simulink model "SF103A_MotRefMdl"  (R2013b)
settings: Solver=FixedStepDiscrete  StartTime=0.0  StopTime=2  FixedStep=.002  RelTol=1e-3
values from neighbouring files (symbols this model uses):
  ARCHGLBPRM_2MILLISEC_SEC_F32 = DataDict.Constant    [SF103A_MotRefMdl_DataDict.m]
  ARCHGLBPRM_2OVERSQRT3_ULS_F32 = DataDict.Constant    [SF103A_MotRefMdl_DataDict.m]
  ARCHGLBPRM_2PI_ULS_F32 = DataDict.Constant    [SF103A_MotRefMdl_DataDict.m]
  ARCHGLBPRM_4OVERSQRT3_ULS_F32 = DataDict.Constant    [SF103A_MotRefMdl_DataDict.m]
  ARCHGLBPRM_5PIOVER4_ULS_F32 = DataDict.Constant    [SF103A_MotRefMdl_DataDict.m]
  ARCHGLBPRM_FLOATZEROTHD_ULS_F32 = DataDict.Constant    [SF103A_MotRefMdl_DataDict.m]
  ARCHGLBPRM_HALFSQRT3_ULS_F32 = DataDict.Constant    [SF103A_MotRefMdl_DataDict.m]
  ARCHGLBPRM_PI_ULS_F32 = DataDict.Constant    [SF103A_MotRefMdl_DataDict.m]
  MotRefMdlCurrDaxBoostGain = DataDict.Calibration    [SF103A_MotRefMdl_DataDict.m]
  MotRefMdlCurrDaxQaxRefDelta = DataDict.Calibration    [SF103A_MotRefMdl_DataDict.m]
  MotRefMdlCurrItrnTolr = DataDict.Calibration    [SF103A_MotRefMdl_DataDict.m]
  MotRefMdlFbCtrlDi = DataDict.Calibration    [SF103A_MotRefMdl_DataDict.m]
  MotRefMdlIvtrDeadTiBrdgVltgSca = DataDict.Calibration    [SF103A_MotRefMdl_DataDict.m]
  MotRefMdlMinCurrItrnLim = DataDict.Calibration    [SF103A_MotRefMdl_DataDict.m]
  MotRefMdlMotCurrDaxMaxSca = DataDict.Calibration    [SF103A_MotRefMdl_DataDict.m]
  MotRefMdlMotVltgDerivtvTiCon = DataDict.Calibration    [SF103A_MotRefMdl_DataDict.m]
  MotRefMdlRefLocnItrnLim = DataDict.Calibration    [SF103A_MotRefMdl_DataDict.m]
  MotRefMdlTqItrnLim = DataDict.Calibration    [SF103A_MotRefMdl_DataDict.m]
  MotRefMdlTqItrnTolr = DataDict.Calibration    [SF103A_MotRefMdl_DataDict.m]
  MotRefMdlVltgModDynCmpEna = DataDict.Calibration    [SF103A_MotRefMdl_DataDict.m]
  MotRefMdlVltgOverRThdSca = DataDict.Calibration    [SF103A_MotRefMdl_DataDict.m]
  SysGlbPrmMotPoleCnt = DataDict.ImprtdCal    [SF103A_MotRefMdl_DataDict.m]
undefined symbols (not defined in the file or in its folder): MotQuad1
libraries: NxtrLim x19, simulink x4, LnrIntrpn x3, Fil x2, NxtrAbslt x2, FixdToFloat x2, FloatToFixd x2, NxtrMath x1
(part 6 of 7)

== system SF103A_MotRefMdl/MotRefMdl/MotRefMdlPer1/DAxisCurrentBoost/If Action Subsystem/If Action Subsystem ==
  note: Rqmts: "BoostAmount"
  note: in requirments module: "VoltageMargin"
  note: Calculate CurrQax
  VRDelta : Inport  RequirementInfo={} %GIDa_629b2140_8cdd_4a04_85a5_53862d241c2d
  InterCalcns : Inport  RequirementInfo={} %GIDa_7ac02062_35f9_44f2_b401_9b07d57448af  Port=2
  CurrDaxMin : Inport  Port=3
  MotTqCmdLimd : Inport  RequirementInfo={} %GIDa_90d50d19_7197_48de_abc9_fa58816f1132  Port=4
  CurrDaxAtPeakTq : Inport  RequirementInfo={} %GIDa_cec05ccb_ae96_4c57_ae99_442dcea898ad  Port=5
  Action Port : ActionPort  ActionType=then
  Abs : Abs  RequirementInfo={'linktype_rmi_doors' '0000bb42 (/E-STEER Core/SubSystem Specifications/Application Functions/SF99/SF103A Motor Reference Model)' '#SF103A_150' 'true' 'REQ:SF103A_150' '' ; 'linktype_rmi_doors' '0000bb42 (/E-STEER Core/SubSystem Specifications/Application Functions/SF99/SF103A Motor Reference Model)' '#SF103A_151' 'true' 'REQ:SF103A_151' '' } %GIDa_3ad1a6bf_5535_4d0e_9aec_c451eb14e8f9
  Add : Sum  RequirementInfo={'linktype_rmi_doors' '0000bb42 (/E-STEER Core/SubSystem Specifications/Application Functions/SF99/SF103A Motor Reference Model)' '#SF103A_154' 'true' 'REQ:SF103A_154' '' } %GIDa_4db111d5_ebda_406f_9d3c_05162b6916bd
  Bus Selector : BusSelector  RequirementInfo={} %GIDa_2a56c463_8bdd_40e7_a9f9_22e566269336  OutputSignals=Ke_VoltPerRadPerSec,RelncTqCoeff_Henry_f32
  Constant1 : Constant  RequirementInfo={'linktype_rmi_doors' '0000bb42 (/E-STEER Core/SubSystem Specifications/Application Functions/SF99/SF103A Motor Reference Model)' '#SF103A_151' 'true' 'REQ:SF103A_151' '' } %GIDa_e17e5b1c_bcf6_46d0_81a3_c3a5d046727d  Value=MotRefMdlCurrDaxBoostGain
  CopyRight2 : Subsystem  Description=|  mask(Copyright Information){none=on}
      | Copyright info block.                                               
      |                                                                     
      | Place copyright information at the top of every subsystem in design.
      mask prompts: none "No parameters"
      mask help: Place copyright information at the top of every subsystem in design.
      mask Display:
      | NxtrConf = 'Nexteer Confidential';
      | 
      | sys = bdroot; %handle for the current model ("system")
      | first = get_param(sys,'Created');
      | first = first(end-3:end);  %year is last four digits
      | 
      | last = get_param(sys,'LastModifiedDate');
      | if isempty(last)
      |     last = datestr(now,'yyyy');
      | else
      |     last = last(end-3:end);
      | end
      | 
      | if strcmp(first,last)
      |     fprintf('%s -- Copyright %s Nexteer',NxtrConf,first)
      | else
      |     fprintf('%s -- %s%s- %s Nexteer',NxtrConf,char(169),first,last)
      | end
  Divide : Product  RequirementInfo={'linktype_rmi_doors' '0000bb42 (/E-STEER Core/SubSystem Specifications/Application Functions/SF99/SF103A Motor Reference Model)' '#SF103A_154' 'true' 'REQ:SF103A_154' '' } %GIDa_ca7e6ec7_86d7_4da8_a1df_b3e0eff68209  Inputs=*/
  FixdToFloat_f32_u16 : FixdToFloat/FixdToFloat_f32_u16  RequirementInfo={'linktype_rmi_doors' '0000bb42 (/E-STEER Core/SubSystem Specifications/Application Functions/SF99/SF103A Motor Reference Model)' '#SF103A_150' 'true' 'REQ:SF103A_150' '' ; 'linktype_rmi_doors' '0000bb42 (/E-STEER Core/SubSystem Specifications/Application Functions/SF99/SF103A Motor Reference Model)' '#SF103A_151' 'true' 'REQ:SF103A_151' '' } %GIDa_b8bb1a83_cb68_4f53_87fe_4f5e4ed3f31f  Param1=15
  FloatToFixd_u16_f32 : FloatToFixd/FloatToFixd_u16_f32  RequirementInfo={'linktype_rmi_doors' '0000bb42 (/E-STEER Core/SubSystem Specifications/Application Functions/SF99/SF103A Motor Reference Model)' '#SF103A_150' 'true' 'REQ:SF103A_150' '' ; 'linktype_rmi_doors' '0000bb42 (/E-STEER Core/SubSystem Specifications/Application Functions/SF99/SF103A Motor Reference Model)' '#SF103A_151' 'true' 'REQ:SF103A_151' '' } %GIDa_bc531b0f_c7c2_47d8_8751_c9c2624b2895  Param1=12
  If : If  RequirementInfo={'linktype_rmi_doors' '0000bb42 (/E-STEER Core/SubSystem Specifications/Application Functions/SF99/SF103A Motor Reference Model)' '#SF103A_153' 'true' 'REQ:SF103A_153' '' } %GIDa_2b3ab8d2_8be4_4128_a6f0_a8ac39a76999  IfExpression=u1
  If Action Subsystem : Subsystem  RequirementInfo={'linktype_rmi_doors' '0000bb42 (/E-STEER Core/SubSystem Specifications/Application Functions/SF99/SF103A Motor Reference Model)' '#SF103A_153' 'true' 'REQ:SF103A_153' '' } %GIDa_e79c30d2_b7e4_4625_82d4_c3d883d510d5  TreatAsAtomicUnit=on
  If Action Subsystem1 : Subsystem  RequirementInfo={'linktype_rmi_doors' '0000bb42 (/E-STEER Core/SubSystem Specifications/Application Functions/SF99/SF103A Motor Reference Model)' '#SF103A_153' 'true' 'REQ:SF103A_153' '' } %GIDa_aa63b104_9695_4c2e_a6b8_97b94259a095  TreatAsAtomicUnit=on
  Merge : Merge
  Product : Product  RequirementInfo={'linktype_rmi_doors' '0000bb42 (/E-STEER Core/SubSystem Specifications/Application Functions/SF99/SF103A Motor Reference Model)' '#SF103A_154' 'true' 'REQ:SF103A_154' '' } %GIDa_fcddbe96_6928_47e1_a12a_56a821b8196f
  Product1 : Product  RequirementInfo={'linktype_rmi_doors' '0000bb42 (/E-STEER Core/SubSystem Specifications/Application Functions/SF99/SF103A Motor Reference Model)' '#SF103A_151' 'true' 'REQ:SF103A_151' '' } %GIDa_b08b78a2_41c7_47f9_9c0f_bbd2ef1a1d8a  Inputs=3  RndMeth=Zero
  Relational Operator : RelationalOperator  RequirementInfo={'linktype_rmi_doors' '0000bb42 (/E-STEER Core/SubSystem Specifications/Application Functions/SF99/SF103A Motor Reference Model)' '#SF103A_153' 'true' 'REQ:SF103A_153' '' } %GIDa_b8fb8f95_bd4b_4329_96ac_0844e2328ed5  OutDataTypeStr=boolean
  Subtract : Sum  RequirementInfo={'linktype_rmi_doors' '0000bb42 (/E-STEER Core/SubSystem Specifications/Application Functions/SF99/SF103A Motor Reference Model)' '#SF103A_152' 'true' 'REQ:SF103A_152' '' } %GIDa_e7614c37_bacf_421b_9d48_2abdeec4ccab  Inputs=+-
  Tq_Characteristic_Table : LnrIntrpn/LnrIntrpn_u16_u16VariXu16VariY  RequirementInfo={'linktype_rmi_doors' '0000bb42 (/E-STEER Core/SubSystem Specifications/Application Functions/SF99/SF103A Motor Reference Model)' '#SF103A_150' 'true' 'REQ:SF103A_150' '' ; 'linktype_rmi_doors' '0000bb42 (/E-STEER Core/SubSystem Specifications/Application Functions/SF99/SF103A Motor Reference Model)' '#SF103A_151' 'true' 'REQ:SF103A_151' '' } %GIDa_dd360f9a_28ce_497a_ac14_fdd325a5e8be  XTbl=MotRefMdlCurrDaxBoostTqScaX  YTbl=MotRefMdlCurrDaxBoostTqScaY
      settings: AttributesFormatString=Lnr ( u16VariX , u16VariY )
  CurrDaxBoostAmnt : Outport  RequirementInfo={} %GIDa_0ceca94c_952e_4fed_8fce_2e415cb9f20e
  CurrDaxBoostd : Outport  RequirementInfo={} %GIDa_8a13dda0_21c7_438d_aecc_2e7f48ec3bef  Port=2
  CurrQaxMin : Outport  RequirementInfo={} %GIDa_d3ca185d_63ed_464a_820c_afb30601f73a  Port=3
  wires:
  Abs/1 -> FloatToFixd_u16_f32/1
  FixdToFloat_f32_u16/1 -> Product1/3
  [TqCmd] -> Abs/1
  Constant1/1 -> Product1/2
  FloatToFixd_u16_f32/1 -> Tq_Characteristic_Table/1
  Tq_Characteristic_Table/1 -> FixdToFloat_f32_u16/1
  Product1/1 -> Subtract/2, CurrDaxBoostAmnt/1
  VRDelta/1 -> Product1/1
  Subtract/1 -> Relational Operator/1, If Action Subsystem/1(BoostProposed)  "BoostProposed"
  CurrDaxMin/1 -> Subtract/1
  MotTqCmdLimd/1 -> [TqCmd]
  InterCalcns/1 -> Bus Selector/1
  Bus Selector/1 -> Add/1  "<Ke_VoltPerRadPerSec>"
  Bus Selector/2 -> Product/1  "<RelncTqCoeff_Henry_f32>"
  Add/1 -> Divide/2
  Product/1 -> Add/2
  Divide/1 -> CurrQaxMin/1
  [TqCmd] -> Divide/1
  If Action Subsystem/1(CurrDaxBoostd) -> Merge/1
  If Action Subsystem1/1(CurrDaxBoostd) -> Merge/2
  Merge/1 -> Product/2, CurrDaxBoostd/1
  If/1 -> If Action Subsystem/Action
  If/2 -> If Action Subsystem1/Action
  Relational Operator/1 -> If/1
  CurrDaxAtPeakTq/1 -> If Action Subsystem1/1(CurrDaxAtPeakTq), Relational Operator/2

== system SF103A_MotRefMdl/MotRefMdl/MotRefMdlPer1/DAxisCurrentBoost/If Action Subsystem/pass_thru ==
  In1 : Inport
  In2 : Inport  Port=2
  In3 : Inport  Port=3
  Action Port : ActionPort  ActionType=else
  Out1 : Outport
  Out2 : Outport  Port=2
  Out3 : Outport  Port=3
  wires:
  In1/1 -> Out1/1
  In2/1 -> Out2/1
  In3/1 -> Out3/1

== system SF103A_MotRefMdl/MotRefMdl/MotRefMdlPer1/FeedforwardVoltage/DynamicTermCalc/CopyRight2 ==

== system SF103A_MotRefMdl/MotRefMdl/MotRefMdlPer1/FeedforwardVoltage/DynamicTermCalc/pass_thru1 ==
  In1 : Inport
  In2 : Inport  Port=2
  Action Port : ActionPort  ActionType=then
  Out1 : Outport
  Out2 : Outport  Port=2
  wires:
  In1/1 -> Out1/1
  In2/1 -> Out2/1

== system SF103A_MotRefMdl/MotRefMdl/MotRefMdlPer1/FeedforwardVoltage/DynamicTermCalc/pass_thru2 ==
  In1 : Inport
  In2 : Inport  Port=2
  Action Port : ActionPort  ActionType=else
  Out1 : Outport
  Out2 : Outport  Port=2
  wires:
  In1/1 -> Out1/1
  In2/1 -> Out2/1

== system SF103A_MotRefMdl/MotRefMdl/MotRefMdlPer1/FeedforwardVoltage/FeedforwardSelection/CopyRight2 ==

== system SF103A_MotRefMdl/MotRefMdl/MotRefMdlPer1/FeedforwardVoltage/FeedforwardSelection/pass_thru1 ==
  In1 : Inport
  In2 : Inport  Port=2
  Action Port : ActionPort  ActionType=then
  Out1 : Outport
  Out2 : Outport  Port=2
  wires:
  In1/1 -> Out1/1
  In2/1 -> Out2/1

== system SF103A_MotRefMdl/MotRefMdl/MotRefMdlPer1/FeedforwardVoltage/FeedforwardSelection/pass_thru2 ==
  In1 : Inport
  In2 : Inport  Port=2
  Action Port : ActionPort  ActionType=else
  Bus Selector : BusSelector  RequirementInfo={'linktype_rmi_doors' '0000bb42 (/E-STEER Core/SubSystem Specifications/Application Functions/SF99/SF103A Motor Reference Model)' '#SF103A_162' 'true' 'REQ:SF103A_162' '' } %GIDa_3a553455_7b79_479b_9241_561868b25559  OutputSignals=EgOverR_Ampr,R_Ohm
  CopyRight2 : Subsystem  Description=|  mask(Copyright Information){none=on}
      | Copyright info block.                                               
      |                                                                     
      | Place copyright information at the top of every subsystem in design.
      mask prompts: none "No parameters"
      mask help: Place copyright information at the top of every subsystem in design.
      mask Display:
      | NxtrConf = 'Nexteer Confidential';
      | 
      | sys = bdroot; %handle for the current model ("system")
      | first = get_param(sys,'Created');
      | first = first(end-3:end);  %year is last four digits
      | 
      | last = get_param(sys,'LastModifiedDate');
      | if isempty(last)
      |     last = datestr(now,'yyyy');
      | else
      |     last = last(end-3:end);
      | end
      | 
      | if strcmp(first,last)
      |     fprintf('%s -- Copyright %s Nexteer',NxtrConf,first)
      | else
      |     fprintf('%s -- %s%s- %s Nexteer',NxtrConf,char(169),first,last)
      | end
  Product : Product  RequirementInfo={'linktype_rmi_doors' '0000bb42 (/E-STEER Core/SubSystem Specifications/Application Functions/SF99/SF103A Motor Reference Model)' '#SF103A_162' 'true' 'REQ:SF103A_162' '' } %GIDa_01f45230_ce72_4e18_a7b2_acaa86327821  RndMeth=Zero
  Out1 : Outport
  Out2 : Outport  Port=2
  wires:
  In1/1 -> Out1/1
  Bus Selector/2 -> Product/2  "<R_Ohm>"
  Bus Selector/1 -> Product/1  "<EgOverR_Ampr>"
  In2/1 -> Bus Selector/1
  Product/1 -> Out2/1

== system SF103A_MotRefMdl/MotRefMdl/MotRefMdlPer1/LocateRef/F_CalcIqCmd_1/CopyRight2 ==

== system SF103A_MotRefMdl/MotRefMdl/MotRefMdlPer1/LocateRef/F_ItoV_1 /CopyRight2 ==

== system SF103A_MotRefMdl/MotRefMdl/MotRefMdlPer1/LocateRef/F_ItoV_2/CopyRight2 ==

== system SF103A_MotRefMdl/MotRefMdl/MotRefMdlPer1/LocateRef/F_VoltTest_1/CopyRight2 ==

== system SF103A_MotRefMdl/MotRefMdl/MotRefMdlPer1/LocateRef/F_VoltTest_1/set_false ==
  In1 : Inport
  Action Port : ActionPort  ActionType=then
  Out1 : Outport
  wires:
  In1/1 -> Out1/1

== system SF103A_MotRefMdl/MotRefMdl/MotRefMdlPer1/LocateRef/F_VoltTest_1/set_true ==
  In1 : Inport
  Action Port : ActionPort  ActionType=else
  Out1 : Outport
  wires:
  In1/1 -> Out1/1

== system SF103A_MotRefMdl/MotRefMdl/MotRefMdlPer1/LocateRef/F_VoltTest_2/CopyRight2 ==

== system SF103A_MotRefMdl/MotRefMdl/MotRefMdlPer1/LocateRef/F_VoltTest_2/set_false ==
  In1 : Inport
  Action Port : ActionPort  ActionType=then
  Out1 : Outport
  wires:
  In1/1 -> Out1/1

== system SF103A_MotRefMdl/MotRefMdl/MotRefMdlPer1/LocateRef/F_VoltTest_2/set_true ==
  In1 : Inport
  Action Port : ActionPort  ActionType=else
  Out1 : Outport
  wires:
  In1/1 -> Out1/1

== system SF103A_MotRefMdl/MotRefMdl/MotRefMdlPer1/LocateRef/for_loop_stuff_here/CopyRight2 ==

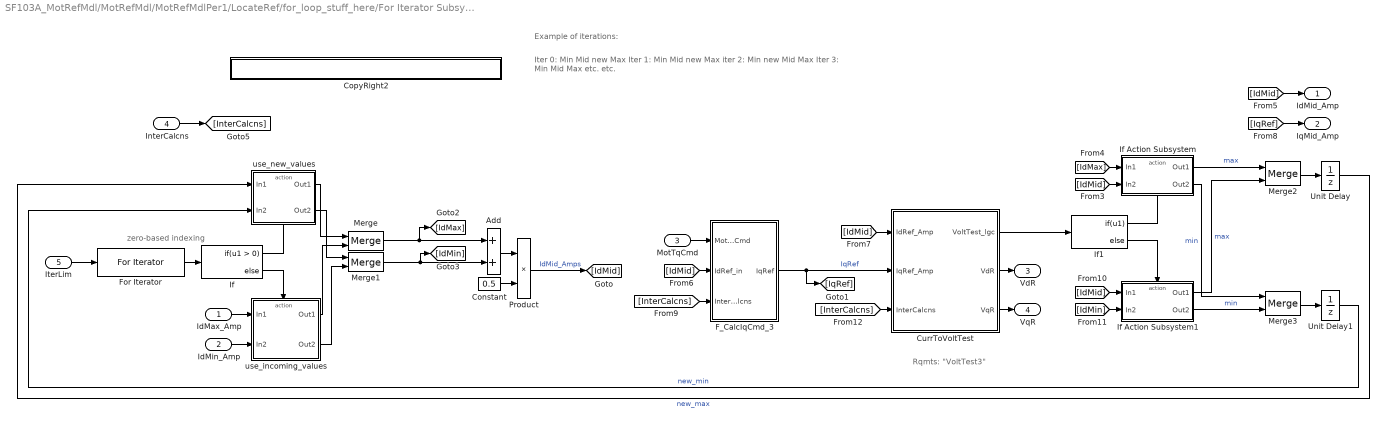
== system SF103A_MotRefMdl/MotRefMdl/MotRefMdlPer1/LocateRef/for_loop_stuff_here/For Iterator Subsystem ==
  note: Rqmts: "VoltTest3"
  note: Example of iterations:
  note: Iter 0:  Min                                        Mid                      new                      Max
      | Iter 1:                                                Min                      Mid        new        Max
      | iter 2:                                                                            Min new Mid        Max
      | Iter 3:                                                                           Min  Mid Max
      | etc.
      | etc.
  note: zero-based indexing
  IdMax_Amp : Inport
  IdMin_Amp : Inport  Port=2
  MotTqCmd : Inport  Port=3
  InterCalcns : Inport  Port=4
  IterLim : Inport  RequirementInfo={} %GIDa_1cf99feb_be11_4d09_9dd2_b31c55a1e7da  Port=5
  Add : Sum  RequirementInfo={'linktype_rmi_doors' '0000bb42 (/E-STEER Core/SubSystem Specifications/Application Functions/SF99/SF103A Motor Reference Model)' '#SF103A_118' 'true' 'REQ:SF103A_118' '' } %GIDa_801a5a52_f315_4cc8_8ec5_019ed326f255
  Constant : Constant  RequirementInfo={'linktype_rmi_doors' '0000bb42 (/E-STEER Core/SubSystem Specifications/Application Functions/SF99/SF103A Motor Reference Model)' '#SF103A_118' 'true' 'REQ:SF103A_118' '' } %GIDa_b46fdda6_5ee2_4848_8152_24810dcb3a94  Value=0.5  OutDataTypeStr=single
  CopyRight2 : Subsystem  Description=|  mask(Copyright Information){none=on}
      | Copyright info block.                                               
      |                                                                     
      | Place copyright information at the top of every subsystem in design.
      mask prompts: none "No parameters"
      mask help: Place copyright information at the top of every subsystem in design.
      mask Display:
      | NxtrConf = 'Nexteer Confidential';
      | 
      | sys = bdroot; %handle for the current model ("system")
      | first = get_param(sys,'Created');
      | first = first(end-3:end);  %year is last four digits
      | 
      | last = get_param(sys,'LastModifiedDate');
      | if isempty(last)
      |     last = datestr(now,'yyyy');
      | else
      |     last = last(end-3:end);
      | end
      | 
      | if strcmp(first,last)
      |     fprintf('%s -- Copyright %s Nexteer',NxtrConf,first)
      | else
      |     fprintf('%s -- %s%s- %s Nexteer',NxtrConf,char(169),first,last)
      | end
  CurrToVoltTest : Subsystem  RequirementInfo={'linktype_rmi_doors' '0000bb42 (/E-STEER Core/SubSystem Specifications/Application Functions/SF99/SF103A Motor Reference Model)' '#SF103A_125' 'true' 'REQ:SF103A_125' '' } %GIDa_afd1848a_308c_456f_8fec_0d556bad692a
  F_CalcIqCmd_3 : Subsystem
  For Iterator : ForIterator  RequirementInfo={'linktype_rmi_doors' '0000bb42 (/E-STEER Core/SubSystem Specifications/Application Functions/SF99/SF103A Motor Reference Model)' '#SF103A_126' 'true' 'REQ:SF103A_126' '' ; 'linktype_rmi_doors' '0000bb42 (/E-STEER Core/SubSystem Specifications/Application Functions/SF99/SF103A Motor Reference Model)' '#SF103A_127' 'true' 'REQ:SF103A_127' '' } %GIDa_240798dc_f011_4595_9579_181698e8b167  IterationSource=external  IterationLimit=MotRefMdlTqItrnLim  IndexMode=Zero-based  IterationVariableDataType=int8
  If : If  RequirementInfo={'linktype_rmi_doors' '0000bb42 (/E-STEER Core/SubSystem Specifications/Application Functions/SF99/SF103A Motor Reference Model)' '#SF103A_126' 'true' 'REQ:SF103A_126' '' ; 'linktype_rmi_doors' '0000bb42 (/E-STEER Core/SubSystem Specifications/Application Functions/SF99/SF103A Motor Reference Model)' '#SF103A_127' 'true' 'REQ:SF103A_127' '' } %GIDa_0c4385fe_0ac3_4314_96e3_cbbd070c57b5
  If Action Subsystem : Subsystem  RequirementInfo={'linktype_rmi_doors' '0000bb42 (/E-STEER Core/SubSystem Specifications/Application Functions/SF99/SF103A Motor Reference Model)' '#SF103A_126' 'true' 'REQ:SF103A_126' '' } %GIDa_cc5a1715_cae9_4ff7_b7f5_7dce45bd5e07  TreatAsAtomicUnit=on
  If Action Subsystem1 : Subsystem  RequirementInfo={'linktype_rmi_doors' '0000bb42 (/E-STEER Core/SubSystem Specifications/Application Functions/SF99/SF103A Motor Reference Model)' '#SF103A_127' 'true' 'REQ:SF103A_127' '' } %GIDa_33229d61_d8d8_448c_8939_4ac7411bbfe6  TreatAsAtomicUnit=on
  If1 : If  RequirementInfo={'linktype_rmi_doors' '0000bb42 (/E-STEER Core/SubSystem Specifications/Application Functions/SF99/SF103A Motor Reference Model)' '#SF103A_126' 'true' 'REQ:SF103A_126' '' ; 'linktype_rmi_doors' '0000bb42 (/E-STEER Core/SubSystem Specifications/Application Functions/SF99/SF103A Motor Reference Model)' '#SF103A_127' 'true' 'REQ:SF103A_127' '' } %GIDa_dc4c98ec_5367_47dd_9994_009a7d002ce4  IfExpression=u1
  Merge : Merge  RequirementInfo={'linktype_rmi_doors' '0000bb42 (/E-STEER Core/SubSystem Specifications/Application Functions/SF99/SF103A Motor Reference Model)' '#SF103A_126' 'true' 'REQ:SF103A_126' '' ; 'linktype_rmi_doors' '0000bb42 (/E-STEER Core/SubSystem Specifications/Application Functions/SF99/SF103A Motor Reference Model)' '#SF103A_127' 'true' 'REQ:SF103A_127' '' } %GIDa_d68afab9_8efc_48e9_af00_8a9c78e21f59
  Merge1 : Merge  RequirementInfo={'linktype_rmi_doors' '0000bb42 (/E-STEER Core/SubSystem Specifications/Application Functions/SF99/SF103A Motor Reference Model)' '#SF103A_126' 'true' 'REQ:SF103A_126' '' ; 'linktype_rmi_doors' '0000bb42 (/E-STEER Core/SubSystem Specifications/Application Functions/SF99/SF103A Motor Reference Model)' '#SF103A_127' 'true' 'REQ:SF103A_127' '' } %GIDa_0e3620e0_3efc_48f8_8171_f5702abde1df
  Merge2 : Merge  RequirementInfo={'linktype_rmi_doors' '0000bb42 (/E-STEER Core/SubSystem Specifications/Application Functions/SF99/SF103A Motor Reference Model)' '#SF103A_126' 'true' 'REQ:SF103A_126' '' } %GIDa_3e05b770_5f19_4125_8232_dc91ee07d6f2
  Merge3 : Merge  RequirementInfo={'linktype_rmi_doors' '0000bb42 (/E-STEER Core/SubSystem Specifications/Application Functions/SF99/SF103A Motor Reference Model)' '#SF103A_127' 'true' 'REQ:SF103A_127' '' } %GIDa_6523f2e4_9eb1_481d_a976_ea57d204ded0
  Product : Product  RequirementInfo={'linktype_rmi_doors' '0000bb42 (/E-STEER Core/SubSystem Specifications/Application Functions/SF99/SF103A Motor Reference Model)' '#SF103A_118' 'true' 'REQ:SF103A_118' '' } %GIDa_4252e675_6653_4a9f_8bc2_a07e04ac2d4a
  Unit Delay : UnitDelay  RequirementInfo={'linktype_rmi_doors' '0000bb42 (/E-STEER Core/SubSystem Specifications/Application Functions/SF99/SF103A Motor Reference Model)' '#SF103A_126' 'true' 'REQ:SF103A_126' '' } %GIDa_f5f1451a_9eea_4a55_998f_2fff27d9d40b  SampleTime=-1
      settings: AttributesFormatString=|
      | Temp Variable
      | No PIM
  Unit Delay1 : UnitDelay  RequirementInfo={'linktype_rmi_doors' '0000bb42 (/E-STEER Core/SubSystem Specifications/Application Functions/SF99/SF103A Motor Reference Model)' '#SF103A_127' 'true' 'REQ:SF103A_127' '' } %GIDa_4fc060ad_847c_4f0f_a937_5f4e973face8  SampleTime=-1
      settings: AttributesFormatString=|
      | Temp Variable
      | No PIM
  use_incoming_values : Subsystem  RequirementInfo={'linktype_rmi_doors' '0000bb42 (/E-STEER Core/SubSystem Specifications/Application Functions/SF99/SF103A Motor Reference Model)' '#SF103A_127' 'true' 'REQ:SF103A_127' '' } %GIDa_3ac2bd99_94e9_4c00_bead_5d2fec2299b9  TreatAsAtomicUnit=on
  use_new_values : Subsystem  RequirementInfo={'linktype_rmi_doors' '0000bb42 (/E-STEER Core/SubSystem Specifications/Application Functions/SF99/SF103A Motor Reference Model)' '#SF103A_126' 'true' 'REQ:SF103A_126' '' } %GIDa_1b33eb44_af9f_4c1f_8219_1430c478da75  TreatAsAtomicUnit=on
  IdMid_Amp : Outport
  IqMid_Amp : Outport  Port=2
  VdR : Outport  Port=3
  VqR : Outport  Port=4
  wires:
  Add/1 -> Product/1
  Merge1/1 -> [IdMin], Add/2
  Merge/1 -> [IdMax], Add/1
  IdMax_Amp/1 -> use_incoming_values/1(In1)
  IdMin_Amp/1 -> use_incoming_values/2(In2)
  Merge2/1 -> Unit Delay/1
  CurrToVoltTest/1(VoltTest_lgc) -> If1/1
  F_CalcIqCmd_3/1(IqRef) -> [IqRef], CurrToVoltTest/2(IqRef_Amp)  "IqRef"
  MotTqCmd/1 -> F_CalcIqCmd_3/1(MotTqCmd)
  Constant/1 -> Product/2
  Product/1 -> [IdMid]  "IdMid_Amps"
  For Iterator/1 -> If/1
  If/2 -> use_incoming_values/Action
  If/1 -> use_new_values/Action
  use_new_values/1(Out1) -> Merge/1
  use_incoming_values/1(Out1) -> Merge/2
  use_new_values/2(Out2) -> Merge1/1
  use_incoming_values/2(Out2) -> Merge1/2
  [IdMid] -> F_CalcIqCmd_3/2(IdRef_in)
  [IdMid] -> IdMid_Amp/1
  InterCalcns/1 -> [InterCalcns]
  [InterCalcns] -> F_CalcIqCmd_3/3(InterCalcns)
  [InterCalcns] -> CurrToVoltTest/3(InterCalcns)
  If1/1 -> If Action Subsystem/Action
  If1/2 -> If Action Subsystem1/Action
  If Action Subsystem/1(Out1) -> Merge2/1  "max"
  If Action Subsystem1/1(Out1) -> Merge2/2  "max"
  [IqRef] -> IqMid_Amp/1
  If Action Subsystem1/2(Out2) -> Merge3/2  "min"
  If Action Subsystem/2(Out2) -> Merge3/1  "min"
  [IdMid] -> If Action Subsystem/2(In2)
  [IdMax] -> If Action Subsystem/1(In1)
  [IdMid] -> If Action Subsystem1/1(In1)
  [IdMin] -> If Action Subsystem1/2(In2)
  Unit Delay/1 -> use_new_values/1(In1)  "new_max"
  Merge3/1 -> Unit Delay1/1
  Unit Delay1/1 -> use_new_values/2(In2)  "new_min"
  IterLim/1 -> For Iterator/1
  CurrToVoltTest/2(VdR) -> VdR/1
  CurrToVoltTest/3(VqR) -> VqR/1
  [IdMid] -> CurrToVoltTest/1(IdRef_Amp)

== system SF103A_MotRefMdl/MotRefMdl/MotRefMdlPer1/LocateTorqueExtremes/CalculateTorque/CopyRight2 ==

== system SF103A_MotRefMdl/MotRefMdl/MotRefMdlPer1/LocateTorqueExtremes/InterpolatePeakTorque/CopyRight2 ==

== system SF103A_MotRefMdl/MotRefMdl/MotRefMdlPer1/LocateTorqueExtremes/InterpolatePeakTorque/F_CalculateTorque ==
  InterCalcns : Inport
  CurrQaxRef : Inport  Port=2
  CurrDaxRef : Inport  Port=3
  Add : Sum
  Bus Selector : BusSelector  OutputSignals=Ke_VoltPerRadPerSec,RelncTqCoeff_Henry_f32
  CopyRight2 : Subsystem  Description=|  mask(Copyright Information){none=on}
      | Copyright info block.                                               
      |                                                                     
      | Place copyright information at the top of every subsystem in design.
      mask prompts: none "No parameters"
      mask help: Place copyright information at the top of every subsystem in design.
      mask Display:
      | NxtrConf = 'Nexteer Confidential';
      | 
      | sys = bdroot; %handle for the current model ("system")
      | first = get_param(sys,'Created');
      | first = first(end-3:end);  %year is last four digits
      | 
      | last = get_param(sys,'LastModifiedDate');
      | if isempty(last)
      |     last = datestr(now,'yyyy');
      | else
      |     last = last(end-3:end);
      | end
      | 
      | if strcmp(first,last)
      |     fprintf('%s -- Copyright %s Nexteer',NxtrConf,first)
      | else
      |     fprintf('%s -- %s%s- %s Nexteer',NxtrConf,char(169),first,last)
      | end
  Product : Product  RndMeth=Zero
  Product1 : Product  RndMeth=Zero
  Torque_MtrNm : Outport
  wires:
  Product1/1 -> Torque_MtrNm/1
  Add/1 -> Product1/1
  CurrDaxRef/1 -> Product/2
  Product/1 -> Add/2
  Bus Selector/2 -> Product/1  "<RelncTqCoeff_Henry_f32>"
  Bus Selector/1 -> Add/1  "<Ke_VoltPerRadPerSec>"
  InterCalcns/1 -> Bus Selector/1
  CurrQaxRef/1 -> Product1/2

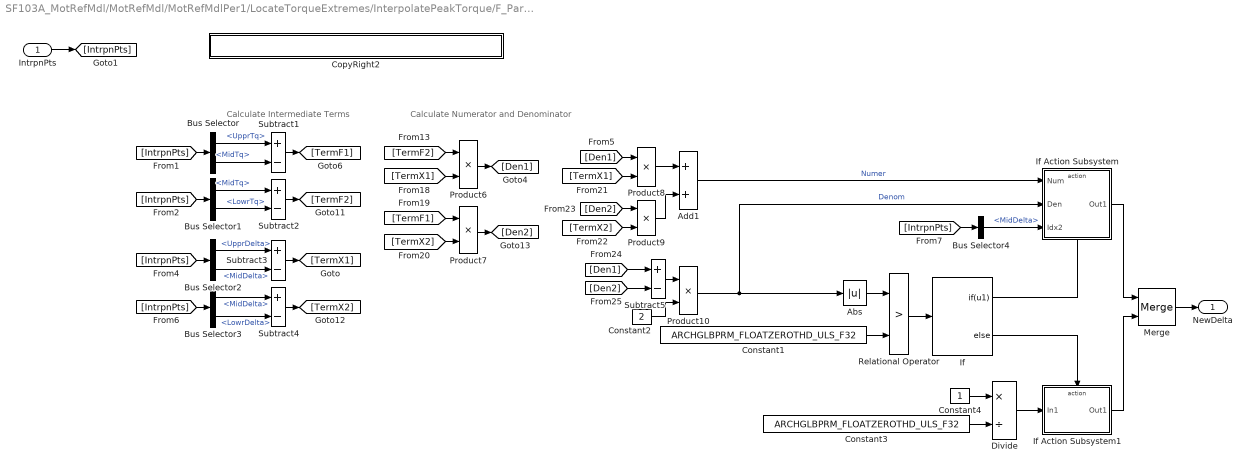
== system SF103A_MotRefMdl/MotRefMdl/MotRefMdlPer1/LocateTorqueExtremes/InterpolatePeakTorque/F_ParabolicInterpolation ==
  note: Calculate Numerator and Denominator
  note: Calculate Intermediate Terms
  IntrpnPts : Inport  RequirementInfo={} %GIDa_3cfb9360_f3a9_4818_b72f_0d6ecc7feaa9
  Abs : Abs  RequirementInfo={'linktype_rmi_doors' '0000bb42 (/E-STEER Core/SubSystem Specifications/Application Functions/SF99/SF103A Motor Reference Model)' '#SF103A_101' 'true' 'REQ:SF103A_101' '' } %GIDa_a9613925_76e1_414d_b339_9c2f25ca70e3
  Add1 : Sum  RequirementInfo={'linktype_rmi_doors' '0000bb42 (/E-STEER Core/SubSystem Specifications/Application Functions/SF99/SF103A Motor Reference Model)' '#SF103A_101' 'true' 'REQ:SF103A_101' '' } %GIDa_5c18b494_af08_4a5d_be70_934d7e0675e9
  Bus Selector : BusSelector  RequirementInfo={} %GIDa_93de9509_a7d0_4f75_8f81_7de43b8aa284  OutputSignals=UpprTq,MidTq
  Bus Selector1 : BusSelector  RequirementInfo={} %GIDa_7a1cad30_9b1b_46dc_984e_690fd0c1598a  OutputSignals=MidTq,LowrTq
  Bus Selector2 : BusSelector  RequirementInfo={} %GIDa_b00839dd_daa8_4156_925c_fc5a7f4de81d  OutputSignals=UpprDelta,MidDelta
  Bus Selector3 : BusSelector  RequirementInfo={} %GIDa_dd2c0c9d_0d94_4d18_b6b6_cae0010b2204  OutputSignals=MidDelta,LowrDelta
  Bus Selector4 : BusSelector  RequirementInfo={} %GIDa_39f453a1_83cd_48de_8e4e_d0f322d1010e  OutputSignals=MidDelta
  Constant1 : Constant  RequirementInfo={'linktype_rmi_doors' '0000bb42 (/E-STEER Core/SubSystem Specifications/Application Functions/SF99/SF103A Motor Reference Model)' '#SF103A_101' 'true' 'REQ:SF103A_101' '' } %GIDa_0a4210c8_e2f7_4887_b479_f5da3b2bf248  Value=ARCHGLBPRM_FLOATZEROTHD_ULS_F32  OutDataTypeStr=single
  Constant2 : Constant  RequirementInfo={'linktype_rmi_doors' '0000bb42 (/E-STEER Core/SubSystem Specifications/Application Functions/SF99/SF103A Motor Reference Model)' '#SF103A_101' 'true' 'REQ:SF103A_101' '' } %GIDa_0fe33e13_e1bd_40f0_b04f_53cbfa19592d  Value=2  OutDataTypeStr=single
  Constant3 : Constant  RequirementInfo={'linktype_rmi_doors' '0000bb42 (/E-STEER Core/SubSystem Specifications/Application Functions/SF99/SF103A Motor Reference Model)' '#SF103A_101' 'true' 'REQ:SF103A_101' '' } %GIDa_8fbb8f60_b251_4ca0_a524_3c91f43e9419  Value=ARCHGLBPRM_FLOATZEROTHD_ULS_F32  OutDataTypeStr=single
  Constant4 : Constant  RequirementInfo={'linktype_rmi_doors' '0000bb42 (/E-STEER Core/SubSystem Specifications/Application Functions/SF99/SF103A Motor Reference Model)' '#SF103A_101' 'true' 'REQ:SF103A_101' '' } %GIDa_b6143dbf_377c_4f79_afdd_6a8010d13014  OutDataTypeStr=single
  CopyRight2 : Subsystem  Description=|  mask(Copyright Information){none=on}
      | Copyright info block.                                               
      |                                                                     
      | Place copyright information at the top of every subsystem in design.
      mask prompts: none "No parameters"
      mask help: Place copyright information at the top of every subsystem in design.
      mask Display:
      | NxtrConf = 'Nexteer Confidential';
      | 
      | sys = bdroot; %handle for the current model ("system")
      | first = get_param(sys,'Created');
      | first = first(end-3:end);  %year is last four digits
      | 
      | last = get_param(sys,'LastModifiedDate');
      | if isempty(last)
      |     last = datestr(now,'yyyy');
      | else
      |     last = last(end-3:end);
      | end
      | 
      | if strcmp(first,last)
      |     fprintf('%s -- Copyright %s Nexteer',NxtrConf,first)
      | else
      |     fprintf('%s -- %s%s- %s Nexteer',NxtrConf,char(169),first,last)
      | end
  Divide : Product  RequirementInfo={'linktype_rmi_doors' '0000bb42 (/E-STEER Core/SubSystem Specifications/Application Functions/SF99/SF103A Motor Reference Model)' '#SF103A_101' 'true' 'REQ:SF103A_101' '' } %GIDa_1bb2cde3_ee3c_40fd_bf34_e395e826b6bc  Inputs=*/
  If : If  RequirementInfo={'linktype_rmi_doors' '0000bb42 (/E-STEER Core/SubSystem Specifications/Application Functions/SF99/SF103A Motor Reference Model)' '#SF103A_101' 'true' 'REQ:SF103A_101' '' } %GIDa_6cb41f5f_7a83_48b4_9a99_9b26b855c6a6  IfExpression=u1
  If Action Subsystem : Subsystem  RequirementInfo={'linktype_rmi_doors' '0000bb42 (/E-STEER Core/SubSystem Specifications/Application Functions/SF99/SF103A Motor Reference Model)' '#SF103A_101' 'true' 'REQ:SF103A_101' '' } %GIDa_5ee13790_179a_4af7_933c_4583aff31551  TreatAsAtomicUnit=on
  If Action Subsystem1 : Subsystem  RequirementInfo={'linktype_rmi_doors' '0000bb42 (/E-STEER Core/SubSystem Specifications/Application Functions/SF99/SF103A Motor Reference Model)' '#SF103A_101' 'true' 'REQ:SF103A_101' '' } %GIDa_6a9e03ce_6bdd_4af7_8129_3d88b4267b2a  TreatAsAtomicUnit=on
  Merge : Merge  RequirementInfo={'linktype_rmi_doors' '0000bb42 (/E-STEER Core/SubSystem Specifications/Application Functions/SF99/SF103A Motor Reference Model)' '#SF103A_101' 'true' 'REQ:SF103A_101' '' } %GIDa_cba85ffc_e36d_4b9a_8942_696bf95c3a9e
  Product10 : Product  RequirementInfo={'linktype_rmi_doors' '0000bb42 (/E-STEER Core/SubSystem Specifications/Application Functions/SF99/SF103A Motor Reference Model)' '#SF103A_101' 'true' 'REQ:SF103A_101' '' } %GIDa_17df0cc6_31b2_4902_8dbb_8ed7bc63bb1c
  Product6 : Product  RequirementInfo={'linktype_rmi_doors' '0000bb42 (/E-STEER Core/SubSystem Specifications/Application Functions/SF99/SF103A Motor Reference Model)' '#SF103A_101' 'true' 'REQ:SF103A_101' '' } %GIDa_b64e116c_b955_4a44_8ab1_dfd17fb9d78e
  Product7 : Product  RequirementInfo={'linktype_rmi_doors' '0000bb42 (/E-STEER Core/SubSystem Specifications/Application Functions/SF99/SF103A Motor Reference Model)' '#SF103A_101' 'true' 'REQ:SF103A_101' '' } %GIDa_7a32fc29_fa8a_4a1b_a674_561745f7434a
  Product8 : Product  RequirementInfo={'linktype_rmi_doors' '0000bb42 (/E-STEER Core/SubSystem Specifications/Application Functions/SF99/SF103A Motor Reference Model)' '#SF103A_101' 'true' 'REQ:SF103A_101' '' } %GIDa_bf709ba6_19a9_4174_8811_a7c57ffe51a4
  Product9 : Product  RequirementInfo={'linktype_rmi_doors' '0000bb42 (/E-STEER Core/SubSystem Specifications/Application Functions/SF99/SF103A Motor Reference Model)' '#SF103A_101' 'true' 'REQ:SF103A_101' '' } %GIDa_e4825d87_aa41_4cd5_8005_4e285c977411
  Relational Operator : RelationalOperator  RequirementInfo={'linktype_rmi_doors' '0000bb42 (/E-STEER Core/SubSystem Specifications/Application Functions/SF99/SF103A Motor Reference Model)' '#SF103A_101' 'true' 'REQ:SF103A_101' '' } %GIDa_c8ed6fda_5911_4294_b3c9_6475a4611c34  Operator=>  OutDataTypeStr=boolean
  Subtract1 : Sum  RequirementInfo={'linktype_rmi_doors' '0000bb42 (/E-STEER Core/SubSystem Specifications/Application Functions/SF99/SF103A Motor Reference Model)' '#SF103A_101' 'true' 'REQ:SF103A_101' '' } %GIDa_ccf6df2d_d0c6_4f84_8a5a_3939a7c4ad54  Inputs=+-
  Subtract2 : Sum  RequirementInfo={'linktype_rmi_doors' '0000bb42 (/E-STEER Core/SubSystem Specifications/Application Functions/SF99/SF103A Motor Reference Model)' '#SF103A_101' 'true' 'REQ:SF103A_101' '' } %GIDa_35ef972f_f2bf_453b_a4a9_d27d8a5c1375  Inputs=+-
  Subtract3 : Sum  RequirementInfo={'linktype_rmi_doors' '0000bb42 (/E-STEER Core/SubSystem Specifications/Application Functions/SF99/SF103A Motor Reference Model)' '#SF103A_101' 'true' 'REQ:SF103A_101' '' } %GIDa_18e6dae4_04b4_4b96_8c89_0050401263ca  Inputs=+-
  Subtract4 : Sum  RequirementInfo={'linktype_rmi_doors' '0000bb42 (/E-STEER Core/SubSystem Specifications/Application Functions/SF99/SF103A Motor Reference Model)' '#SF103A_101' 'true' 'REQ:SF103A_101' '' } %GIDa_e21bf7a3_795d_46e3_aa86_778fa88d2588  Inputs=+-
  Subtract5 : Sum  RequirementInfo={'linktype_rmi_doors' '0000bb42 (/E-STEER Core/SubSystem Specifications/Application Functions/SF99/SF103A Motor Reference Model)' '#SF103A_101' 'true' 'REQ:SF103A_101' '' } %GIDa_d18a91e0_2c64_4271_8783_f3e2d703c3cd  Inputs=+-
  NewDelta : Outport  RequirementInfo={} %GIDa_46c36f57_13be_4170_ae8f_61aafc35e215
  wires:
  Subtract1/1 -> [TermF1]
  Subtract2/1 -> [TermF2]
  Subtract3/1 -> [TermX1]
  Subtract4/1 -> [TermX2]
  [TermF2] -> Product6/1
  [TermX1] -> Product6/2
  Product6/1 -> [Den1]
  [TermF1] -> Product7/1
  [TermX2] -> Product7/2
  Product7/1 -> [Den2]
  [Den1] -> Product8/1
  [TermX1] -> Product8/2
  [Den2] -> Product9/1
  [TermX2] -> Product9/2
  Product8/1 -> Add1/1
  Product9/1 -> Add1/2
  Add1/1 -> If Action Subsystem/1(Num)  "Numer"
  [Den1] -> Subtract5/1
  [Den2] -> Subtract5/2
  Subtract5/1 -> Product10/1
  Constant2/1 -> Product10/2
  Product10/1 -> Abs/1, If Action Subsystem/2(Den)  "Denom"
  Constant1/1 -> Relational Operator/2
  Abs/1 -> Relational Operator/1
  Relational Operator/1 -> If/1
  If/1 -> If Action Subsystem/Action
  Constant3/1 -> Divide/2
  Constant4/1 -> Divide/1
  Divide/1 -> If Action Subsystem1/1(In1)
  If/2 -> If Action Subsystem1/Action
  Merge/1 -> NewDelta/1
  If Action Subsystem/1(Out1) -> Merge/1
  If Action Subsystem1/1(Out1) -> Merge/2
  [IntrpnPts] -> Bus Selector/1
  IntrpnPts/1 -> [IntrpnPts]
  Bus Selector/1 -> Subtract1/1  "<UpprTq>"
  Bus Selector/2 -> Subtract1/2  "<MidTq>"
  [IntrpnPts] -> Bus Selector1/1
  Bus Selector1/1 -> Subtract2/1  "<MidTq>"
  Bus Selector1/2 -> Subtract2/2  "<LowrTq>"
  [IntrpnPts] -> Bus Selector2/1
  Bus Selector2/1 -> Subtract3/1  "<UpprDelta>"
  Bus Selector2/2 -> Subtract3/2  "<MidDelta>"
  [IntrpnPts] -> Bus Selector3/1
  Bus Selector3/1 -> Subtract4/1  "<MidDelta>"
  Bus Selector3/2 -> Subtract4/2  "<LowrDelta>"
  [IntrpnPts] -> Bus Selector4/1
  Bus Selector4/1 -> If Action Subsystem/3(Idx2)  "<MidDelta>"

== system SF103A_MotRefMdl/MotRefMdl/MotRefMdlPer1/LocateTorqueExtremes/InterpolatePeakTorque/F_VSinCosToIdIq ==
  InterCalcns : Inport
  SinDelta : Inport  Port=2
  CosDelta : Inport  Port=3
  Add : Sum
  Bus Selector2 : BusSelector  OutputSignals=ReacncDaxOverR,VovrRovrZ_Ampr,EgOverROverZ_Ampr,ReacncQaxOverR,VltgOverR_Ampr
  CopyRight2 : Subsystem  Description=|  mask(Copyright Information){none=on}
      | Copyright info block.                                               
      |                                                                     
      | Place copyright information at the top of every subsystem in design.
      mask prompts: none "No parameters"
      mask help: Place copyright information at the top of every subsystem in design.
      mask Display:
      | NxtrConf = 'Nexteer Confidential';
      | 
      | sys = bdroot; %handle for the current model ("system")
      | first = get_param(sys,'Created');
      | first = first(end-3:end);  %year is last four digits
      | 
      | last = get_param(sys,'LastModifiedDate');
      | if isempty(last)
      |     last = datestr(now,'yyyy');
      | else
      |     last = last(end-3:end);
      | end
      | 
      | if strcmp(first,last)
      |     fprintf('%s -- Copyright %s Nexteer',NxtrConf,first)
      | else
      |     fprintf('%s -- %s%s- %s Nexteer',NxtrConf,char(169),first,last)
      | end
  Product{,1..3} (4 alike) : Product  RndMeth=Zero
  Subtract : Sum  Inputs=+-
  Subtract1 : Sum  Inputs=+-
  CurrQaxRef : Outport
  CurrDaxRef : Outport  Port=2
  wires:
  Subtract1/1 -> CurrDaxRef/1  "IdRef_Amp"
  Product3/1 -> Subtract1/2
  Product2/1 -> Subtract1/1
  Subtract/1 -> CurrQaxRef/1, Product2/1  "IqRef_Amp"
  Product1/1 -> Subtract/1
  SinDelta/1 -> Product3/2, Product/1
  Bus Selector2/5 -> Product3/1  "<VltgOverR_Ampr>"
  Bus Selector2/4 -> Product2/2  "<ReacncQaxOverR>"
  Bus Selector2/3 -> Subtract/2  "<EgOverROverZ_Ampr>"
  Bus Selector2/1 -> Product/2  "<ReacncDaxOverR>"
  Bus Selector2/2 -> Product1/2  "<VovrRovrZ_Ampr>"
  InterCalcns/1 -> Bus Selector2/1
  Add/1 -> Product1/1
  CosDelta/1 -> Add/1
  Product/1 -> Add/2

== system SF103A_MotRefMdl/MotRefMdl/MotRefMdlPer1/LocateTorqueExtremes/InterpolatePeakTorque/Initialize_Points ==
  In1 : Inport
  Action Port : ActionPort  ActionType=then
  Signal Conversion : SignalConversion
  Out1 : Outport
  wires:
  In1/1 -> Signal Conversion/1
  Signal Conversion/1 -> Out1/1

== system SF103A_MotRefMdl/MotRefMdl/MotRefMdlPer1/LocateTorqueExtremes/InterpolatePeakTorque/Refine_Higher ==
  OldPts : Inport
  NewDelta : Inport  Port=2
  NewTq : Inport  Port=3
  Action Port : ActionPort  ActionType=else
  Bus Creator : BusCreator  Inputs=6
  Bus Selector : BusSelector  OutputSignals=MidDelta,MidTq,LowrDelta,LowrTq
  CopyRight2 : Subsystem  Description=|  mask(Copyright Information){none=on}
      | Copyright info block.                                               
      |                                                                     
      | Place copyright information at the top of every subsystem in design.
      mask prompts: none "No parameters"
      mask help: Place copyright information at the top of every subsystem in design.
      mask Display:
      | NxtrConf = 'Nexteer Confidential';
      | 
      | sys = bdroot; %handle for the current model ("system")
      | first = get_param(sys,'Created');
      | first = first(end-3:end);  %year is last four digits
      | 
      | last = get_param(sys,'LastModifiedDate');
      | if isempty(last)
      |     last = datestr(now,'yyyy');
      | else
      |     last = last(end-3:end);
      | end
      | 
      | if strcmp(first,last)
      |     fprintf('%s -- Copyright %s Nexteer',NxtrConf,first)
      | else
      |     fprintf('%s -- %s%s- %s Nexteer',NxtrConf,char(169),first,last)
      | end
  Data Type Conversion : DataTypeConversion
  Data Type Conversion1 : DataTypeConversion
  Signal Conversion : SignalConversion
  Out1 : Outport
  wires:
  NewDelta/1 -> Bus Creator/3  "MidDelta"
  NewTq/1 -> Bus Creator/4  "MidTq"
  Bus Creator/1 -> Signal Conversion/1
  OldPts/1 -> Bus Selector/1
  Data Type Conversion/1 -> Bus Creator/1  "UpprDelta"
  Data Type Conversion1/1 -> Bus Creator/2  "UpprTq"
  Signal Conversion/1 -> Out1/1
  Bus Selector/1 -> Data Type Conversion/1  "<MidDelta>"
  Bus Selector/2 -> Data Type Conversion1/1  "<MidTq>"
  Bus Selector/3 -> Bus Creator/5  "<LowrDelta>"
  Bus Selector/4 -> Bus Creator/6  "<LowrTq>"

== system SF103A_MotRefMdl/MotRefMdl/MotRefMdlPer1/LocateTorqueExtremes/InterpolatePeakTorque/Refine_Lower ==
  OldPts : Inport
  NewDelta : Inport  Port=2
  NewTq : Inport  Port=3
  Action Port : ActionPort  ActionType=then
  Bus Creator : BusCreator  Inputs=6
  Bus Selector : BusSelector  OutputSignals=UpprDelta,UpprTq,MidDelta,MidTq
  CopyRight2 : Subsystem  Description=|  mask(Copyright Information){none=on}
      | Copyright info block.                                               
      |                                                                     
      | Place copyright information at the top of every subsystem in design.
      mask prompts: none "No parameters"
      mask help: Place copyright information at the top of every subsystem in design.
      mask Display:
      | NxtrConf = 'Nexteer Confidential';
      | 
      | sys = bdroot; %handle for the current model ("system")
      | first = get_param(sys,'Created');
      | first = first(end-3:end);  %year is last four digits
      | 
      | last = get_param(sys,'LastModifiedDate');
      | if isempty(last)
      |     last = datestr(now,'yyyy');
      | else
      |     last = last(end-3:end);
      | end
      | 
      | if strcmp(first,last)
      |     fprintf('%s -- Copyright %s Nexteer',NxtrConf,first)
      | else
      |     fprintf('%s -- %s%s- %s Nexteer',NxtrConf,char(169),first,last)
      | end
  Data Type Conversion : DataTypeConversion
  Data Type Conversion1 : DataTypeConversion
  Signal Conversion : SignalConversion
  Out1 : Outport
  wires:
  Bus Selector/1 -> Bus Creator/1  "<UpprDelta>"
  Bus Selector/2 -> Bus Creator/2  "<UpprTq>"
  Bus Selector/3 -> Data Type Conversion1/1  "<MidDelta>"
  NewDelta/1 -> Bus Creator/3  "MidDelta"
  NewTq/1 -> Bus Creator/4  "MidTq"
  Bus Creator/1 -> Signal Conversion/1
  OldPts/1 -> Bus Selector/1
  Signal Conversion/1 -> Out1/1
  Bus Selector/4 -> Data Type Conversion/1  "<MidTq>"
  Data Type Conversion1/1 -> Bus Creator/5  "LowrDelta"
  Data Type Conversion/1 -> Bus Creator/6  "LowrTq"

== system SF103A_MotRefMdl/MotRefMdl/MotRefMdlPer1/LocateTorqueExtremes/InterpolatePeakTorque/Use_Refined_Points ==
  In1 : Inport
  Action Port : ActionPort  ActionType=else
  Signal Conversion : SignalConversion
  Out1 : Outport
  wires:
  In1/1 -> Signal Conversion/1
  Signal Conversion/1 -> Out1/1

== system SF103A_MotRefMdl/MotRefMdl/MotRefMdlPer1/LocateTorqueExtremes/Negative/CopyRight2 ==

== system SF103A_MotRefMdl/MotRefMdl/MotRefMdlPer1/LocateTorqueExtremes/Negative/For Iterator Subsystem ==
  note: NOTE: Zero-based indexing
  note: No PIM needed.  This is inside a
      | FOR loop, so the data does not need to
      | be remembered across calls to Per1 runnable.
  note: NOTE: Zero-based indexing
  TqAry : Inport
  Constant : Constant  Value=0  OutDataTypeStr=uint8
  CopyRight2 : Subsystem  Description=|  mask(Copyright Information){none=on}
      | Copyright info block.                                               
      |                                                                     
      | Place copyright information at the top of every subsystem in design.
      mask prompts: none "No parameters"
      mask help: Place copyright information at the top of every subsystem in design.
      mask Display:
      | NxtrConf = 'Nexteer Confidential';
      | 
      | sys = bdroot; %handle for the current model ("system")
      | first = get_param(sys,'Created');
      | first = first(end-3:end);  %year is last four digits
      | 
      | last = get_param(sys,'LastModifiedDate');
      | if isempty(last)
      |     last = datestr(now,'yyyy');
      | else
      |     last = last(end-3:end);
      | end
      | 
      | if strcmp(first,last)
      |     fprintf('%s -- Copyright %s Nexteer',NxtrConf,first)
      | else
      |     fprintf('%s -- %s%s- %s Nexteer',NxtrConf,char(169),first,last)
      | end
  Data Type Conversion : DataTypeConversion  OutDataTypeStr=uint8
  For Iterator : ForIterator  IterationSource=external  IterationLimit=8  IndexMode=Zero-based  IterationVariableDataType=int8
      settings: AttributesFormatString=ItrnLim: %<IterationLimit>
  Found_New_Min : Subsystem  TreatAsAtomicUnit=on
  If1 : If  NumInputs=2  IfExpression=u1 | u2  ShowElse=off
  Relational Operator : RelationalOperator  Operator=<=  OutDataTypeStr=boolean
  Relational Operator1 : RelationalOperator  Operator===  OutDataTypeStr=boolean
  Selector : Selector  IndexMode=Zero-based  InputPortWidth=8  IndexOptions=Starting index (port)  Indices=[1 3]  OutputSizes=1
  Unit Delay1 : UnitDelay  SampleTime=-1
  Width : Width
  IdxSt : Outport  InitialOutput=0
      settings: AttributesFormatString=IC = %<InitialOutput>
  wires:
  Width/1 -> For Iterator/1
  TqAry/1 -> Selector/1, Width/1
  [ItrnNr] -> Selector/2
  For Iterator/1 -> Data Type Conversion/1
  Found_New_Min/1(IdxSt) -> IdxSt/1
  Selector/1 -> Relational Operator/1, [Tq]
  [Tq] -> Found_New_Min/2(Tq)
  [ItrnNr] -> Found_New_Min/1(Idx)
  Data Type Conversion/1 -> Relational Operator1/1, [ItrnNr]
  If1/1 -> Found_New_Min/Action
  Found_New_Min/2(TqSt) -> Unit Delay1/1  "TqSt"
  Constant/1 -> Relational Operator1/2
  Relational Operator1/1 -> If1/1
  Relational Operator/1 -> If1/2
  Unit Delay1/1 -> Relational Operator/2

== system SF103A_MotRefMdl/MotRefMdl/MotRefMdlPer1/LocateTorqueExtremes/Positive/CopyRight2 ==

== system SF103A_MotRefMdl/MotRefMdl/MotRefMdlPer1/LocateTorqueExtremes/Positive/For Iterator Subsystem ==
  note: No PIM needed.  This is inside a
      | FOR loop, so the data does not need to
      | be remembered across calls to Per1 runnable.
  note: NOTE: Zero-based indexing
  note: NOTE: Zero-based indexing
  TqAry : Inport
  Constant : Constant  Value=0  OutDataTypeStr=uint8
  CopyRight2 : Subsystem  Description=|  mask(Copyright Information){none=on}
      | Copyright info block.                                               
      |                                                                     
      | Place copyright information at the top of every subsystem in design.
      mask prompts: none "No parameters"
      mask help: Place copyright information at the top of every subsystem in design.
      mask Display:
      | NxtrConf = 'Nexteer Confidential';
      | 
      | sys = bdroot; %handle for the current model ("system")
      | first = get_param(sys,'Created');
      | first = first(end-3:end);  %year is last four digits
      | 
      | last = get_param(sys,'LastModifiedDate');
      | if isempty(last)
      |     last = datestr(now,'yyyy');
      | else
      |     last = last(end-3:end);
      | end
      | 
      | if strcmp(first,last)
      |     fprintf('%s -- Copyright %s Nexteer',NxtrConf,first)
      | else
      |     fprintf('%s -- %s%s- %s Nexteer',NxtrConf,char(169),first,last)
      | end
  Data Type Conversion : DataTypeConversion  OutDataTypeStr=uint8
  For Iterator : ForIterator  IterationSource=external  IterationLimit=8  IndexMode=Zero-based  IterationVariableDataType=int8
      settings: AttributesFormatString=ItrnLim: %<IterationLimit>
  Found_New_Max : Subsystem  TreatAsAtomicUnit=on
  If : If  NumInputs=2  IfExpression=u1 | u2  ShowElse=off
  Relational Operator : RelationalOperator  OutDataTypeStr=boolean
  Relational Operator1 : RelationalOperator  Operator===  OutDataTypeStr=boolean
  Selector : Selector  IndexMode=Zero-based  InputPortWidth=8  IndexOptions=Starting index (port)  Indices=[1 3]  OutputSizes=1
  Unit Delay : UnitDelay  SampleTime=-1
  Width : Width
  IdxSt : Outport  InitialOutput=0
      settings: AttributesFormatString=IC = %<InitialOutput>
  wires:
  Width/1 -> For Iterator/1
  Found_New_Max/1(IdxSt) -> IdxSt/1
  TqAry/1 -> Selector/1, Width/1
  [ItrnNr] -> Selector/2
  For Iterator/1 -> Data Type Conversion/1
  Selector/1 -> Relational Operator/1, [Tq]
  [Tq] -> Found_New_Max/2(Tq)
  [ItrnNr] -> Found_New_Max/1(Idx)
  Data Type Conversion/1 -> Relational Operator1/1, [ItrnNr]
  If/1 -> Found_New_Max/Action
  Found_New_Max/2(TqSt) -> Unit Delay/1  "TqSt"
  Constant/1 -> Relational Operator1/2
  Relational Operator1/1 -> If/1
  Relational Operator/1 -> If/2
  Unit Delay/1 -> Relational Operator/2

== system SF103A_MotRefMdl/MotRefMdl/MotRefMdlPer1/LocateTorqueExtremes/WrapBracketAngles/CopyRight2 ==
